simulink model "pr21"  (R2019b)
settings: Solver=VariableStepAuto  StartTime=0.0  StopTime=30.00  RelTol=1e-3
settings Model: Creator=Gonzalo Sanz  LastModifiedBy=Gonzalo Sanz

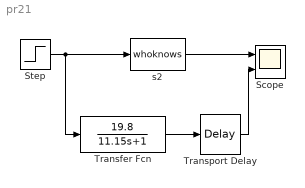
== system pr21 ==
  Scope : Scope  NumInputPorts=2
  Step : Step  SampleTime=0
  Transfer Fcn : TransferFcn  Numerator=[19.8]  Denominator=[11.15 1]
  Transport Delay : TransportDelay  DelayTime=3.2
  s2 : M-S-Function  FunctionName=whoknows  Parameters=L, P1, P2, T, R  mask{L=7, P1=0, P2=7, T=1, R=0}
      mask prompts: L "Laboratorio"; P1 "Primer digito del Puesto"; P2 "Segundo digito del Puesto"; T "Tipo de Planta"; R "Ruido"
      mask Display: disp('Sistema')
  wires:
  s2/1 -> Scope/1
  Step/1 -> Transfer Fcn/1, s2/1
  Transfer Fcn/1 -> Transport Delay/1
  Transport Delay/1 -> Scope/2
